simulink model "sim_Exp81"  (R2019a)
settings: Solver=VariableStepAuto  StartTime=0.0  StopTime=10.0  RelTol=1e-3
undefined symbols (not defined in the file): GP_den, GP_num
settings Model: Creator=sgxgong4  LastModifiedBy=sgxgong4

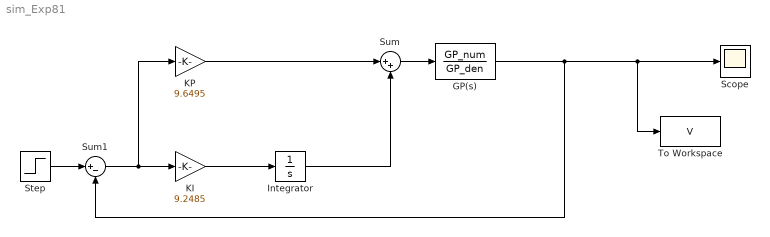
== system sim_Exp81 ==
  GP(s) : TransferFcn  Numerator=GP_num  Denominator=GP_den
  Integrator : Integrator
  KI : Gain  Gain=9.2485
  KP : Gain  Gain=9.6495
  Scope : Scope
  Step : Step  Time=0  SampleTime=0
  Sum : Sum  Inputs=|++
  Sum1 : Sum  Inputs=|+-
  To Workspace : ToWorkspace  VariableName=V  SaveFormat=Structure With Time  SampleTime=-1
  wires:
  KI/1 -> Integrator/1
  KP/1 -> Sum/1
  Integrator/1 -> Sum/2
  Sum1/1 -> KP/1, KI/1
  Step/1 -> Sum1/1
  Sum/1 -> GP(s)/1
  GP(s)/1 -> Sum1/2, To Workspace/1, Scope/1
